simulink model "MX28"  (R2014b)
settings: Solver=FixedStepDiscrete  StartTime=0.0  StopTime=10.0  RelTol=1e-3
values from neighbouring files (symbols this model uses):
  MX28_amplifier = MX28_supply_voltage/1024    (= 0.01171875)    [MX28_init.m]
  MX28_init_position = pi    (= 3.14159265359)    [MX28_init.m]
  MX28_Kc = 8e-3    (= 0.008)    [MX28_init.m]
  MX28_Kd = 1/8    (= 0.125)    [MX28_init.m]
  MX28_Ki = 1/1024    (= 0.0009765625)    [MX28_init.m]
  MX28_Kp = 1/4    (= 0.25)    [MX28_init.m]
  MX28_Kv = 9.926e-3    (= 0.009926)    [MX28_init.m]
  MX28_position_gain = 4096 / 2 / pi    (= 651.898646904)    [MX28_init.m]
  MX28_reduction = 192.6    [MX28_init.m]
  MX28_resistor = 8.3    [MX28_init.m]
  MX28_speed_gain = 1024 / 8    (= 128)    [MX28_init.m]
  MX28_Te = 1/1000    (= 0.001)    [MX28_init.m]
libraries: simulink x4, simulink_extras x1
settings Model: Creator=florent  LastModifiedBy=florent
settings OptimizationCC: InlineParams=on
settings DebuggingCC: ParameterPrecisionLossMsg=none  StateNameClashWarn=warning

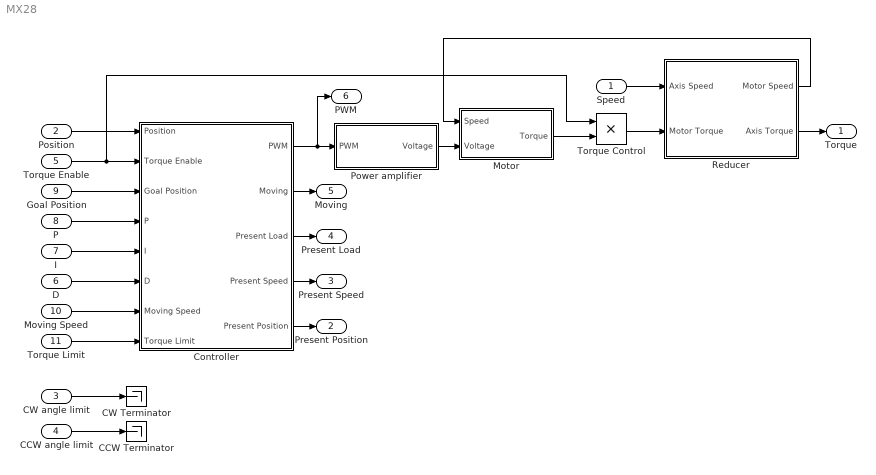
== system MX28 ==
  Speed : Inport
  Position : Inport  Port=2
  CW angle limit : Inport  Port=3  OutDataTypeStr=int16
  CCW angle limit : Inport  Port=4  OutDataTypeStr=int16
  Torque Enable : Inport  Port=5  OutDataTypeStr=boolean
  D : Inport  Port=6  OutDataTypeStr=uint8
  I : Inport  Port=7  OutDataTypeStr=uint8
  P : Inport  Port=8  OutDataTypeStr=uint8
  Goal Position : Inport  Port=9
  Moving Speed : Inport  Port=10  OutDataTypeStr=int16
  Torque Limit : Inport  Port=11  OutDataTypeStr=int16
  CCW Terminator : Terminator
  CW Terminator : Terminator
  Controller : Subsystem  TreatAsAtomicUnit=on
  Motor : Subsystem
  Power amplifier : Subsystem  TreatAsAtomicUnit=on
  Reducer : Subsystem
  Torque Control : Product
  Torque : Outport
  Present Position : Outport  Port=2
  Present Speed : Outport  Port=3
  Present Load : Outport  Port=4
  Moving : Outport  Port=5
  PWM : Outport  Port=6
  wires:
  Position/1 -> Controller/1(Position)
  Reducer/1(Motor Speed) -> Motor/1(Speed)
  Controller/1(PWM) -> Power amplifier/1(PWM), PWM/1
  Speed/1 -> Reducer/1(Axis Speed)
  Reducer/2(Axis Torque) -> Torque/1
  Torque Control/1 -> Reducer/2(Motor Torque)
  Power amplifier/1(Voltage) -> Motor/2(Voltage)
  Controller/2(Moving) -> Moving/1
  Controller/3(Present Load) -> Present Load/1
  Controller/4(Present Speed) -> Present Speed/1
  Controller/5(Present Position) -> Present Position/1
  Torque Enable/1 -> Torque Control/1, Controller/2(Torque Enable)
  Goal Position/1 -> Controller/3(Goal Position)
  P/1 -> Controller/4(P)
  I/1 -> Controller/5(I)
  D/1 -> Controller/6(D)
  Torque Limit/1 -> Controller/8(Torque Limit)
  Moving Speed/1 -> Controller/7(Moving Speed)
  Motor/1(Torque) -> Torque Control/2
  CW angle limit/1 -> CW Terminator/1
  CCW angle limit/1 -> CCW Terminator/1

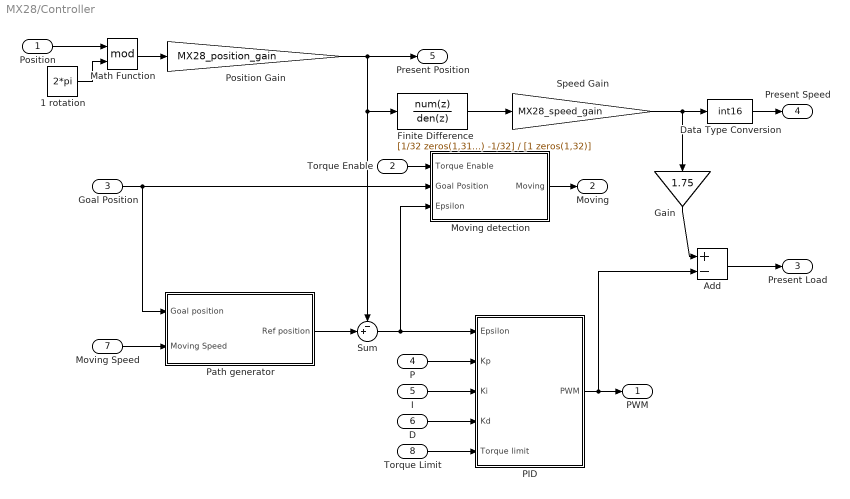
== system MX28/Controller ==
  Position : Inport
  Torque Enable : Inport  Port=2
  Goal Position : Inport  Port=3  OutDataTypeStr=int16
  P : Inport  Port=4
  I : Inport  Port=5
  D : Inport  Port=6
  Moving Speed : Inport  Port=7
  Torque Limit : Inport  Port=8
  1 rotation : Constant  Value=2*pi
  Add : Sum  Inputs=+-
  Data Type Conversion : DataTypeConversion  OutDataTypeStr=int16
  Finite Difference : DiscreteTransferFcn  Numerator=[1/32 zeros(1,31) -1/32]  Denominator=[1 zeros(1,32)]  InitialStates=MX28_init_position * MX28_position_gain  a0EqualsOne=on
  Gain : Gain  Gain=1.75  OutDataTypeStr=int16
  Math Function : Math  Operator=mod  SaturateOnIntegerOverflow=on
  Moving detection : Subsystem  TreatAsAtomicUnit=on
  PID : Subsystem  TreatAsAtomicUnit=on  SystemSampleTime=0.001
  Path generator : Subsystem  TreatAsAtomicUnit=on
  Position Gain : Gain  Gain=MX28_position_gain  OutMin=0  OutMax=4095  OutDataTypeStr=int16  RndMeth=Zero  SampleTime=MX28_Te  SaturateOnIntegerOverflow=on
  Speed Gain : Gain  Gain=MX28_speed_gain  OutDataTypeStr=double
  Sum : Sum  Inputs=-+|  AccumDataTypeStr=double  OutMin=-4095  OutMax=4095  OutDataTypeStr=int16  SaturateOnIntegerOverflow=on
  PWM : Outport
  Moving : Outport  Port=2
  Present Load : Outport  Port=3
  Present Speed : Outport  Port=4
  Present Position : Outport  Port=5
  wires:
  Position Gain/1 -> Present Position/1, Finite Difference/1, Sum/1
  Math Function/1 -> Position Gain/1
  Position/1 -> Math Function/1
  1 rotation/1 -> Math Function/2
  Sum/1 -> PID/1(Epsilon), Moving detection/3(Epsilon)
  PID/1(PWM) -> Add/2, PWM/1
  P/1 -> PID/2(Kp)
  I/1 -> PID/3(Ki)
  D/1 -> PID/4(Kd)
  Moving detection/1(Moving) -> Moving/1
  Goal Position/1 -> Path generator/1(Goal position), Moving detection/2(Goal Position)
  Torque Enable/1 -> Moving detection/1(Torque Enable)
  Torque Limit/1 -> PID/5(Torque limit)
  Speed Gain/1 -> Data Type Conversion/1, Gain/1
  Finite Difference/1 -> Speed Gain/1
  Path generator/1(Ref position) -> Sum/2
  Moving Speed/1 -> Path generator/2(Moving Speed)
  Add/1 -> Present Load/1
  Gain/1 -> Add/1
  Data Type Conversion/1 -> Present Speed/1

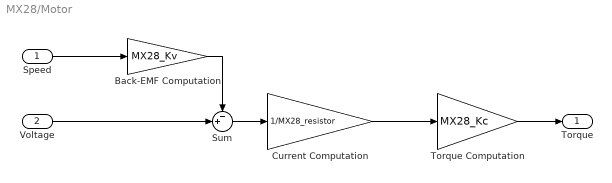
== system MX28/Motor ==
  Speed : Inport
  Voltage : Inport  Port=2
  Back-EMF Computation : Gain  Gain=MX28_Kv
  Current Computation : Gain  Gain=1/MX28_resistor
  Sum : Sum  Inputs=-+|
  Torque Computation : Gain  Gain=MX28_Kc
  Torque : Outport
  wires:
  Sum/1 -> Current Computation/1
  Voltage/1 -> Sum/2
  Back-EMF Computation/1 -> Sum/1
  Speed/1 -> Back-EMF Computation/1
  Torque Computation/1 -> Torque/1
  Current Computation/1 -> Torque Computation/1

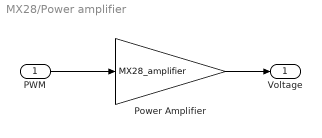
== system MX28/Power amplifier ==
  PWM : Inport
  Power Amplifier : Gain  Gain=MX28_amplifier  OutDataTypeStr=double
  Voltage : Outport
  wires:
  PWM/1 -> Power Amplifier/1
  Power Amplifier/1 -> Voltage/1

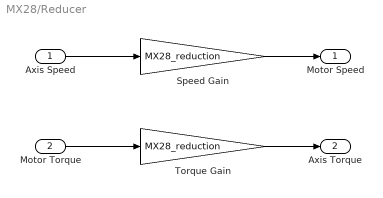
== system MX28/Reducer ==
  Axis Speed : Inport
  Motor Torque : Inport  Port=2
  Speed Gain : Gain  Gain=MX28_reduction
  Torque Gain : Gain  Gain=MX28_reduction
  Motor Speed : Outport
  Axis Torque : Outport  Port=2
  wires:
  Torque Gain/1 -> Axis Torque/1
  Motor Torque/1 -> Torque Gain/1
  Axis Speed/1 -> Speed Gain/1
  Speed Gain/1 -> Motor Speed/1

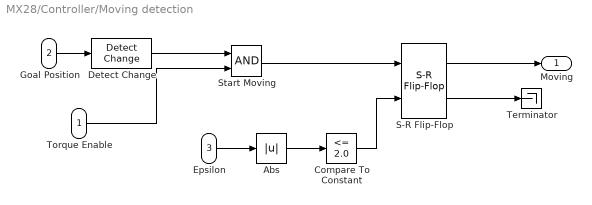
== system MX28/Controller/Moving detection ==
  Torque Enable : Inport
  Goal Position : Inport  Port=2
  Epsilon : Inport  Port=3
  Abs : Abs
  Compare To Constant : simulink/Logic and Bit Operations/Compare To Constant  relop=<=  const=2.0  OutDataTypeStr=boolean
  Detect Change : simulink/Logic and Bit Operations/Detect Change  vinit=0  InputProcessing=Inherited  OutDataTypeStr=boolean
  S-R Flip-Flop : simulink_extras/Flip Flops/S-R Flip-Flop  initial_condition=0
  Start Moving : Logic  AllPortsSameDT=off  OutDataTypeStr=boolean
  Terminator : Terminator
  Moving : Outport
  wires:
  Detect Change/1 -> Start Moving/1
  Compare To Constant/1 -> S-R Flip-Flop/2
  Goal Position/1 -> Detect Change/1
  Torque Enable/1 -> Start Moving/2
  Epsilon/1 -> Abs/1
  Start Moving/1 -> S-R Flip-Flop/1
  S-R Flip-Flop/1 -> Moving/1
  Abs/1 -> Compare To Constant/1
  S-R Flip-Flop/2 -> Terminator/1

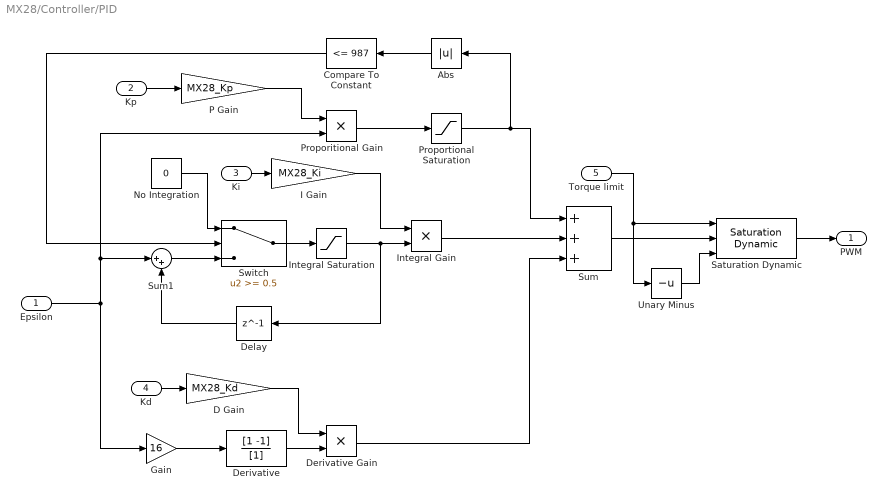
== system MX28/Controller/PID ==
  Epsilon : Inport
  Kp : Inport  Port=2
  Ki : Inport  Port=3
  Kd : Inport  Port=4
  Torque limit : Inport  Port=5
  Abs : Abs
  Compare To Constant : simulink/Logic and Bit Operations/Compare To Constant  relop=<=  const=987  OutDataTypeStr=boolean
  D Gain : Gain  Gain=MX28_Kd  OutDataTypeStr=double
  Delay : Delay  DelayLength=1  SampleTime=MX28_Te
  Derivative : DiscreteFilter  Numerator=[1 -1]  Denominator=[1]
  Derivative Gain : Product
  Gain : Gain  Gain=16
  I Gain : Gain  Gain=MX28_Ki  OutDataTypeStr=double
  Integral Gain : Product
  Integral Saturation : Saturate  UpperLimit=30690  LowerLimit=-30690
  No Integration : Constant  Value=0
  P Gain : Gain  Gain=MX28_Kp  OutDataTypeStr=double
  Proporitional Gain : Product
  Proportional Saturation : Saturate  UpperLimit=987  LowerLimit=-987
  Saturation Dynamic : simulink/Discontinuities/Saturation Dynamic  OutMin=[]  OutMax=[]  OutDataTypeStr=Inherit: Same as second input  OutDataType=fixdt(1, 16)  OutScaling=2^-10  DoSatur=off
  Sum : Sum  Inputs=+++  OutDataTypeStr=int16  SaturateOnIntegerOverflow=on
  Sum1 : Sum  Inputs=|++
  Switch : Switch  Threshold=0.5
  Unary Minus : UnaryMinus
  PWM : Outport
  wires:
  Epsilon/1 -> Proporitional Gain/2, Sum1/1, Gain/1
  Derivative Gain/1 -> Sum/3
  Kp/1 -> P Gain/1
  Ki/1 -> I Gain/1
  Integral Gain/1 -> Sum/2
  Kd/1 -> D Gain/1
  Derivative/1 -> Derivative Gain/2
  No Integration/1 -> Switch/1
  Switch/1 -> Integral Saturation/1
  Sum1/1 -> Switch/3
  Proporitional Gain/1 -> Proportional Saturation/1
  Proportional Saturation/1 -> Abs/1, Sum/1
  Integral Saturation/1 -> Delay/1, Integral Gain/2
  Delay/1 -> Sum1/2
  Gain/1 -> Derivative/1
  Compare To Constant/1 -> Switch/2
  Abs/1 -> Compare To Constant/1
  P Gain/1 -> Proporitional Gain/1
  I Gain/1 -> Integral Gain/1
  D Gain/1 -> Derivative Gain/1
  Saturation Dynamic/1 -> PWM/1
  Sum/1 -> Saturation Dynamic/2
  Torque limit/1 -> Unary Minus/1, Saturation Dynamic/1
  Unary Minus/1 -> Saturation Dynamic/3

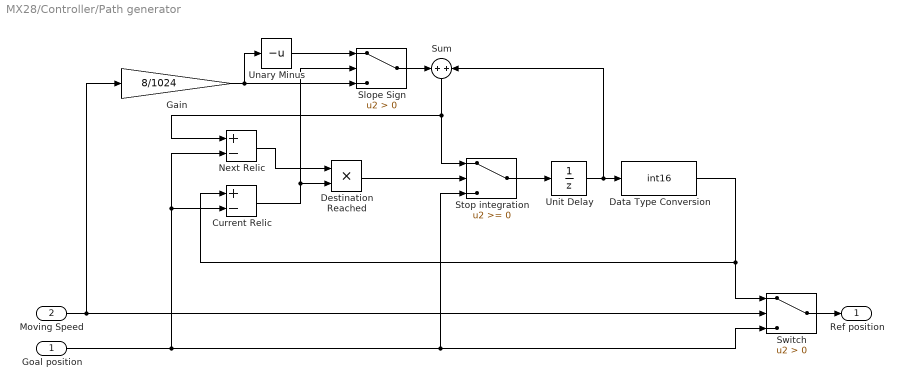
== system MX28/Controller/Path generator ==
  Goal position : Inport
  Moving Speed : Inport  Port=2
  "Current Relic " : Sum  Inputs=+-
  Data Type Conversion : DataTypeConversion  OutDataTypeStr=int16
  Destination Reached : Product
  Gain : Gain  Gain=8/1024  ParamDataTypeStr=double
  Next Relic : Sum  Inputs=+-
  Slope Sign : Switch  Criteria=u2 > Threshold
  Stop integration : Switch
  Sum : Sum  Inputs=+|+
  Switch : Switch  Criteria=u2 > Threshold
  Unary Minus : UnaryMinus
  Unit Delay : UnitDelay  InitialCondition=MX28_init_position * MX28_position_gain  SampleTime=-1
  Ref position : Outport
  wires:
  Moving Speed/1 -> Gain/1, Switch/2
  Goal position/1 -> Stop integration/3, Switch/3, "Current Relic "/2, Next Relic/2
  Switch/1 -> Ref position/1
  Gain/1 -> Slope Sign/3, Unary Minus/1
  Slope Sign/1 -> Sum/1
  Sum/1 -> Stop integration/1, Next Relic/1
  "Current Relic "/1 -> Destination Reached/2, Slope Sign/2
  Next Relic/1 -> Destination Reached/1
  Destination Reached/1 -> Stop integration/2
  Data Type Conversion/1 -> "Current Relic "/1, Switch/1
  Unary Minus/1 -> Slope Sign/1
  Unit Delay/1 -> Data Type Conversion/1, Sum/2
  Stop integration/1 -> Unit Delay/1
